simulink model "Simulation_2_joint_manipulator"  (R2023a)
settings: Solver=VariableStepAuto  StartTime=0.0  StopTime=10  RelTol=1e-3
libraries: simulink_extras x2
settings Model: PacingRate=1000  Creator=ACCENT  LastModifiedBy=ACCENT

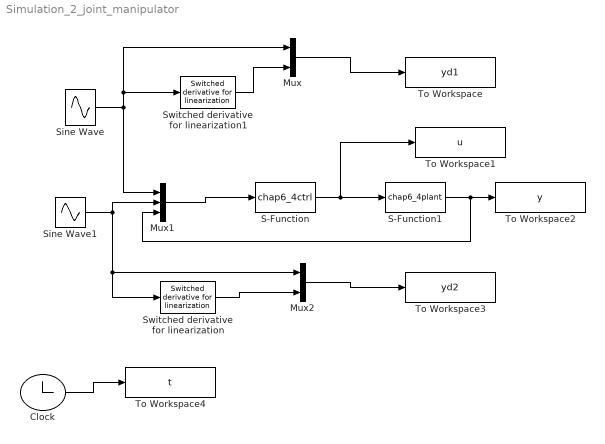
== system Simulation_2_joint_manipulator ==
  Clock : Clock
  Mux : Mux  Inputs=2
  Mux1 : Mux  Inputs=3
  Mux2 : Mux  Inputs=2
  S-Function : S-Function  FunctionName=chap6_4ctrl  SFunctionDeploymentMode=off  EnableBusSupport=off
  S-Function1 : S-Function  FunctionName=chap6_4plant  SFunctionDeploymentMode=off  EnableBusSupport=off
  Sine Wave : Sin  Frequency=2  SampleTime=0
  Sine Wave1 : Sin  Frequency=2  SampleTime=0
  Switched derivative for linearization : simulink_extras/Linearization/Switched derivative for linearization  switchVal=0  derivConst=100
  Switched derivative for linearization1 : simulink_extras/Linearization/Switched derivative for linearization  switchVal=0  derivConst=100
  To Workspace : ToWorkspace  VariableName=yd1  SampleTime=-1
  To Workspace1 : ToWorkspace  VariableName=u  SampleTime=-1
  To Workspace2 : ToWorkspace  VariableName=y  SampleTime=-1
  To Workspace3 : ToWorkspace  VariableName=yd2  SampleTime=-1
  To Workspace4 : ToWorkspace  VariableName=t  SampleTime=-1
  wires:
  Sine Wave/1 -> Switched derivative for linearization1/1, Mux/1, Mux1/1
  Switched derivative for linearization1/1 -> Mux/2
  Mux/1 -> To Workspace/1
  Sine Wave1/1 -> Switched derivative for linearization/1, Mux2/1, Mux1/2
  Mux1/1 -> S-Function/1
  S-Function/1 -> To Workspace1/1, S-Function1/1
  Switched derivative for linearization/1 -> Mux2/2
  Mux2/1 -> To Workspace3/1
  Clock/1 -> To Workspace4/1
  S-Function1/1 -> Mux1/3, To Workspace2/1
